simulink model "pendulum"  (R2019a)
settings: Solver=VariableStepAuto  StartTime=0.0  StopTime=20  RelTol=1e-3
settings Model: Creator=TAGS Administrator  LastModifiedBy=TAGS Administrator

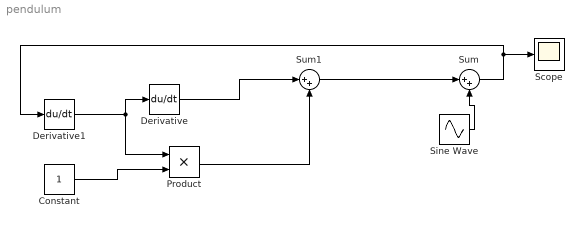
== system pendulum ==
  Constant : Constant
  Derivative : Derivative  CoefficientInTFapproximation=4
  Derivative1 : Derivative  CoefficientInTFapproximation=0
  Product : Product
  Scope : Scope
  Sine Wave : Sin  SampleTime=0
  Sum : Sum  Inputs=|++
  Sum1 : Sum  Inputs=|++
  wires:
  Product/1 -> Sum1/2
  Sum1/1 -> Sum/1
  Sine Wave/1 -> Sum/2
  Constant/1 -> Product/2
  Derivative1/1 -> Derivative/1, Product/1
  Sum/1 -> Scope/1, Derivative1/1
  Derivative/1 -> Sum1/1
